simulink model "nomoto_model"  (R2014a)
settings: Solver=ode45  StartTime=0.0  StopTime=tstop  RelTol=1e-3
values from neighbouring files (symbols this model uses):
  d_c = 15 * (pi/180)    (= 0.261799387799)    [run.m]
  K = c_f(1) / d_c    [run.m]
  T = 1 / c_f(2)    [run.m]
  tsamp = 10    [run.m]
settings Model: CovSFcnEnable=on  Creator=patrickf  LastModifiedBy=Hwk
settings OptimizationCC: SimCompilerOptimization=off
settings DebuggingCC: MergeDetectMultiDrivingBlocksExec=error  SolverPrmCheckMsg=none  FrameProcessingCompatibilityMsg=error
settings RTWCC: RTWCompilerOptimization=off

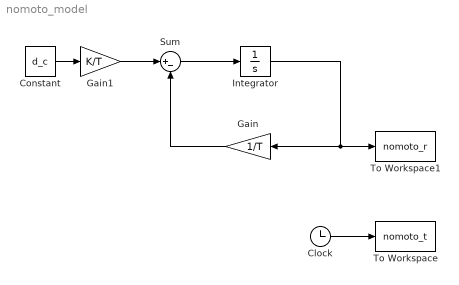
== system nomoto_model ==
  Clock : Clock
  Constant : Constant  Value=d_c
  Gain : Gain  Gain=1/T
  Gain1 : Gain  Gain=K/T
  Integrator : Integrator
  Sum : Sum  Inputs=|+-
  To Workspace : ToWorkspace  VariableName=nomoto_t  SampleTime=tsamp
  To Workspace1 : ToWorkspace  VariableName=nomoto_r  SampleTime=tsamp
  wires:
  Sum/1 -> Integrator/1
  Integrator/1 -> To Workspace1/1, Gain/1
  Gain/1 -> Sum/2
  Constant/1 -> Gain1/1
  Gain1/1 -> Sum/1
  Clock/1 -> To Workspace/1
